simulink model "B_double_simu_3states"  (R2015a)
settings: Solver=ode45  SolverMode=SingleTasking  StartTime=0.0  StopTime=500  RelTol=1e-3
values from neighbouring files (symbols this model uses):
  A = -1*[-1/L2 ... (first row only)    [ett_slap.m]    (also in linearss_circle.m = -1*[-1/L4 1/L3 0; states_5_linearss.m = -1*[0 1 0 0 0; tva_slap.m = -1*[-1/L3 1/L2)
  B = -1*[1/L1]'    [ett_slap.m]    (also in linearss_circle.m = -1*[0 0 1/L1]'; states_5_linearss.m = -1*[0 0 0 0 1/L1]'; tva_slap.m = -1*[0 1/L1]')
  C = eye(1)    [ett_slap.m]    (also in linearss_circle.m = eye(3); states_5_linearss.m = eye(5); tva_slap.m = eye(2))
  D = zeros(1,1)    [ett_slap.m]    (also in linearss_circle.m = zeros(3,1); states_5_linearss.m = zeros(5,1); tva_slap.m = zeros(2,1))
  Xd = [phi1e]    [ett_slap.m]    (also in linearss_circle.m = [phi3e;phi2e;phi1e]; tva_slap.m = [phi2e;phi1e])
undefined symbols (not defined in the file or in its folder): K
libraries: simulink x5, simulink_extras x3
settings Model: CovSFcnEnable=off  Creator=marcus  LastModifiedBy=marcus
settings OptimizationCC: BlockReduction=off  BooleanDataType=off
settings DebuggingCC: SaveWithParameterizedLinksMsg=none  UnderspecifiedInitializationDetection=Classic  MergeDetectMultiDrivingBlocksExec=none  SignalResolutionControl=TryResolveAllWithWarning
settings HardwareCC: TargetUnknown=on

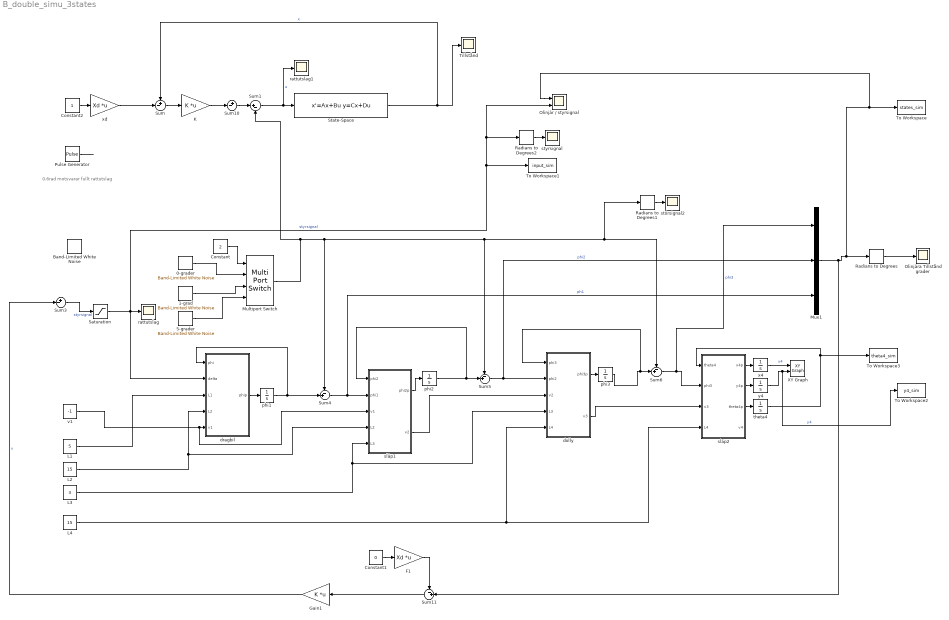
== system B_double_simu_3states ==
  note: 0.6rad motsvarar fullt rattutslag
  0-grader : simulink/Sources/Band-Limited White Noise  Cov=[0.00000]  Ts=0.1  seed=[1]
  1-grad : simulink/Sources/Band-Limited White Noise  Cov=[0.000005]  Ts=0.1  seed=[1]
  5-grader : simulink/Sources/Band-Limited White Noise  Cov=[0.00009]  Ts=0.1  seed=[1]
  Band-Limited White Noise : simulink/Sources/Band-Limited White Noise  Cov=[0.0001]  Ts=0.1  seed=[23341]
  Constant : Constant  Value=2  VectorParams1D=off  SampleTime=-1
  Constant1 : Constant  Value=0
  Constant2 : Constant
  F1 : Gain  Gain=Xd  Multiplication=Matrix(K*u)
  Gain1 : Gain  Gain=K  Multiplication=Matrix(K*u)
  K : Gain  Gain=K  Multiplication=Matrix(K*u)
  L1 : Constant  Value=5  SampleTime=1
  L2 : Constant  Value=15  SampleTime=1
  L3 : Constant  Value=3  SampleTime=1
  L4 : Constant  Value=15  SampleTime=1
  Multiport Switch : MultiPortSwitch
  Mux1 : Mux  Inputs=3
  Olinjär / styrsignal : Scope  NumInputPorts=2
      settings: TickLabels=on  ShowLegends=on  YMin=-5~-0.2  YMax=2~0.4
  Olinjära Tillstånd grader : Scope
      settings: ShowLegends=on
  Pulse Generator : DiscretePulseGenerator  PulseType=Time based  Amplitude=0.1  Period=1000  PhaseDelay=5
  Radians to Degrees : simulink_extras/Transformations/Radians to Degrees
  Radians to Degrees1 : simulink_extras/Transformations/Radians to Degrees
  Radians to Degrees2 : simulink_extras/Transformations/Radians to Degrees
  Saturation : Saturate  UpperLimit=0.7  LowerLimit=-0.7
  State-Space : StateSpace  A=A  B=B  C=C  D=D  X0=0  ContinuousStateAttributes={'a', 'b', 'c'}
  Sum : Sum  Inputs=+-|
  Sum1 : Sum  Inputs=|+-
  Sum10 : Sum  Inputs=+-|
  Sum{4..6,11} (4 alike) : Sum  Inputs=-+|
  Sum3 : Sum  Inputs=+-|
  Tillstånd : Scope
      settings: ShowLegends=on  YMin=0  YMax=1  SaveName=ScopeData4
  To Workspace : ToWorkspace  VariableName=states_sim  SampleTime=-1
      settings: Save2DSignal=2-D array (concatenate along first dimension)
  To Workspace1 : ToWorkspace  VariableName=input_sim  SampleTime=-1
      settings: Save2DSignal=2-D array (concatenate along first dimension)
  To Workspace2 : ToWorkspace  VariableName=y4_sim  SampleTime=-1
      settings: Save2DSignal=2-D array (concatenate along first dimension)
  To Workspace3 : ToWorkspace  VariableName=theta4_sim  SampleTime=-1
      settings: Save2DSignal=2-D array (concatenate along first dimension)
  XY Graph : simulink/Sinks/XY Graph  xmin=-150  xmax=100  ymin=-200  ymax=50  st=10
  dolly : MATLAB Function  TreatAsAtomicUnit=on
  dragbil : MATLAB Function  TreatAsAtomicUnit=on
  phi1 : Integrator
  phi2 : Integrator
  phi3 : Integrator
  rattutslag : Scope
      settings: ShowLegends=on  SaveName=ScopeData2
  rattutslag1 : Scope
      settings: ShowLegends=on  SaveName=ScopeData3
  släp1 : MATLAB Function  TreatAsAtomicUnit=on
  släp2 : MATLAB Function  TreatAsAtomicUnit=on
  styrsignal : Scope
      settings: ShowLegends=on  SaveName=ScopeData6
  störsignal2 : Scope
      settings: ShowLegends=on  SaveName=ScopeData5
  theta4 : Integrator
  v1 : Constant  Value=-1  SampleTime=1
  x4 : Integrator
  "xd " : Gain  Gain=Xd  Multiplication=Matrix(K*u)
  y4 : Integrator
  wires:
  dolly/1(phi3p) -> phi3/1
  släp1/1(phi2p) -> phi2/1
  dragbil/1(phip) -> phi1/1
  släp2/3(theta4p) -> theta4/1
  v1/1 -> släp1/3(v1), dragbil/5(v1)
  L2/1 -> dragbil/4(L2), släp1/4(L2)
  L1/1 -> dragbil/3(L1)
  Sum1/1 -> rattutslag1/1, State-Space/1  "u"
  dolly/2(v3) -> släp2/3(v3)
  släp1/2(v2) -> dolly/3(v2)
  theta4/1 -> To Workspace3/1, släp2/1(theta4)
  L3/1 -> dolly/4(L3), släp1/5(L3)
  L4/1 -> dolly/5(L4), släp2/4(L4)
  Gain1/1 -> Sum3/2  "v"
  Multiport Switch/1 -> Sum1/2, Radians to Degrees1/1, Sum6/1, Sum5/1, Sum4/1
  Sum5/1 -> Mux1/2, dolly/2(phi2)  "phi2"
  Sum6/1 -> Mux1/1, släp2/2(phi3)  "phi3"
  Sum4/1 -> Mux1/3, släp1/2(phi1)  "ph1"
  Saturation/1 -> rattutslag/1, To Workspace1/1, Olinjär / styrsignal/2, Radians to Degrees2/1, dragbil/2(delta)  "styrsignal"
  Pulse Generator/1 -> ?
  phi3/1 -> dolly/1(phi3), Sum6/2
  phi2/1 -> släp1/1(phi2), Sum5/2
  phi1/1 -> Sum4/2, dragbil/1(phi)
  State-Space/1 -> Tillstånd/1, Sum/1  "x"
  "xd "/1 -> Sum/2
  Sum10/1 -> Sum1/1
  Sum/1 -> K/1
  K/1 -> Sum10/2
  Sum11/1 -> Gain1/1
  Constant1/1 -> F1/1
  Constant2/1 -> "xd "/1
  Radians to Degrees/1 -> Olinjära Tillstånd grader/1
  släp2/1(x4p) -> x4/1
  x4/1 -> XY Graph/1  "x4"
  släp2/2(y4p) -> y4/1
  y4/1 -> To Workspace2/1, XY Graph/2  "y4"
  Radians to Degrees1/1 -> störsignal2/1
  Radians to Degrees2/1 -> styrsignal/1
  Sum3/1 -> Saturation/1  "styrsignal"
  F1/1 -> Sum11/1
  Mux1/1 -> Olinjär / styrsignal/1, To Workspace/1, Radians to Degrees/1, Sum11/2
  0-grader/1 -> Multiport Switch/2
  5-grader/1 -> Multiport Switch/4
  1-grad/1 -> Multiport Switch/3
  Constant/1 -> Multiport Switch/1

== matlab function B_double_simu_3states/släp1 ==
  data: phi2 input; phi1 input; v1 input; phi2p output; L2 input; L3 input; v2 output
function [phi2p,v2]= fcn(phi2,phi1,v1,L2,L3)
%#codegen


v2 = v1*cos(phi1);
phi2p = v2*(tan(phi1)/L2-sin(phi2)/L3);

== matlab function B_double_simu_3states/dragbil ==
  data: phi input; delta input; phip output; L1 input; L2 input; v1 input
function phip = fcn(phi,delta,L1,L2,v1)
%#codegen

phip = v1*(tan(delta)/L1-sin(phi)/L2);

== matlab function B_double_simu_3states/dolly ==
  data: phi3 input; phi2 input; v2 input; L3 input; phi3p output; L4 input; v3 output
function [phi3p,v3]= fcn(phi3,phi2,v2,L3,L4)
%#codegen

v3 = v2*cos(phi2);
phi3p = v3*(tan(phi2)/L3-sin(phi3)/L4);

== matlab function B_double_simu_3states/släp2 ==
  data: theta4 input; phi3 input; v3 input; x4p output; L4 input; y4p output; theta4p output; v4 output
function [x4p,y4p,theta4p,v4]= fcn(theta4,phi3,v3,L4)
%#codegen

v4 = v3*cos(phi3);
theta4p=v4*tan(phi3)/L4;
x4p=v4*cos(theta4);
y4p=v4*sin(theta4);
